simulink model "model_2023"  (R2023a)
settings: Solver=VariableStepAuto  StartTime=0.0  StopTime=100  RelTol=1e-3
settings Model: Creator=ian20030201  LastModifiedBy=ian20030201

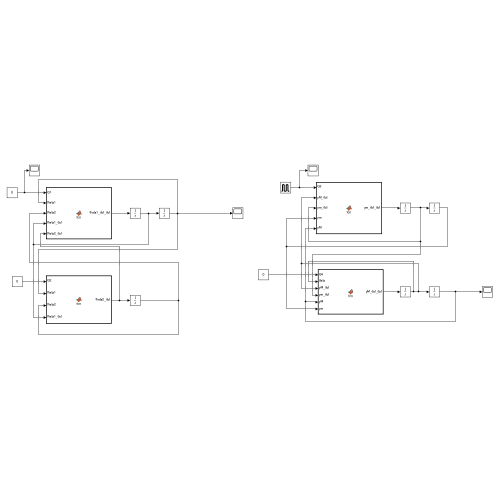
[thumbnail: Simulink's stored preview of the top-level diagram]
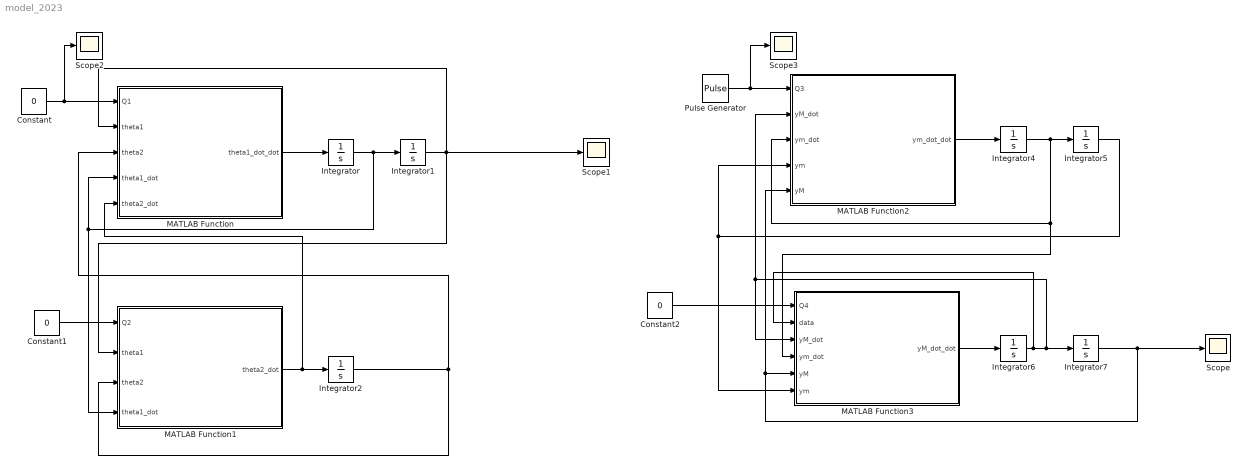
== system model_2023 ==
  Constant : Constant  Value=0
  Constant1 : Constant  Value=0
  Constant2 : Constant  Value=0
  Integrator{,1..2,4..7} (7 alike) : Integrator
  MATLAB Function : MATLAB Function  TreatAsAtomicUnit=on
  MATLAB Function1 : MATLAB Function  TreatAsAtomicUnit=on
  MATLAB Function2 : MATLAB Function  TreatAsAtomicUnit=on
  MATLAB Function3 : MATLAB Function  TreatAsAtomicUnit=on
  Pulse Generator : DiscretePulseGenerator  PulseType=Time based  Amplitude=20000  Period=100  PulseWidth=5  PhaseDelay=10
  Scope{,1..3} (4 alike) : Scope
  wires:
  MATLAB Function/1(theta1_dot_dot) -> Integrator/1
  Integrator/1 -> MATLAB Function1/4(theta1_dot), MATLAB Function/4(theta1_dot), Integrator1/1
  MATLAB Function1/1(theta2_dot) -> MATLAB Function/5(theta2_dot), Integrator2/1
  MATLAB Function2/1(ym_dot_dot) -> Integrator4/1
  Integrator4/1 -> MATLAB Function3/4(ym_dot), MATLAB Function2/3(ym_dot), Integrator5/1
  MATLAB Function3/1(yM_dot_dot) -> Integrator6/1
  Integrator6/1 -> MATLAB Function3/2(data), MATLAB Function3/3(yM_dot), MATLAB Function2/2(yM_dot), Integrator7/1
  Integrator2/1 -> MATLAB Function1/3(theta2), MATLAB Function/3(theta2)
  Integrator1/1 -> Scope1/1, MATLAB Function1/2(theta1), MATLAB Function/2(theta1)
  Integrator5/1 -> MATLAB Function3/6(ym), MATLAB Function2/4(ym)
  Integrator7/1 -> Scope/1, MATLAB Function2/5(yM), MATLAB Function3/5(yM)
  Constant/1 -> Scope2/1, MATLAB Function/1(Q1)
  Constant1/1 -> MATLAB Function1/1(Q2)
  Pulse Generator/1 -> Scope3/1, MATLAB Function2/1(Q3)
  Constant2/1 -> MATLAB Function3/1(Q4)

== matlab function model_2023/MATLAB Function1 ==
  data: Q2 input; theta2_dot output; theta1 input; theta2 input; theta1_dot input
function theta2_dot = fcn(Q2, theta1, theta2, theta1_dot)
c4 = 0.1;
l = 5;
k4 = 1000;
top = Q2 + c4 * l^2 * (cos(theta2) - cos(theta1 + theta2)) * cos(theta1 + theta2) * theta1_dot + k4 * l^2 * (sin(theta1 + 2*theta2) - 0.5 * sin(2*theta1 + 2*theta2) - 0.5 * sin(2*theta2));
bottom = c4 * l^2 * (cos(theta1 + theta2) - cos(theta2))^2;
bottom = 1;
theta2_dot = top / bottom;

== matlab function model_2023/MATLAB Function ==
  data: Q1 input; theta1_dot_dot output; theta1 input; theta2 input; theta1_dot input; theta2_dot input
function theta1_dot_dot = fcn(Q1, theta1, theta2, theta1_dot, theta2_dot)
c4 = 0.1;
l = 5;
m1 = 1000; m3 = 1000;
k1 = 1000; k3 = 1000; k4 = 1000;
g = 9.81;
top = Q1 - c4 * l^2 * (cos(theta1 + theta2))^2 * theta1_dot - c4 * l^2 * (cos(theta1 + theta2))^2 * theta2_dot + c4 * l^2 * (cos(theta1 + theta2)) * cos(theta2) * theta2_dot;
top = top - g * l * m1 * cos(theta1) + g * l * m3 * cos(theta1) - 0.5 * k1 * l^2 * sin(2*theta1) - 0.5 * k3 * l^2 * sin(2*theta1) - 0.5 * k4 * l^2 * sin(2*theta1) + 2 * theta2 + k4 * l^2 * sin(theta2) * cos(theta1 + theta2);
bottom = l^2 * (m1 + m3);

theta1_dot_dot = top / bottom;

== matlab function model_2023/MATLAB Function2 ==
  data: Q3 input; ym_dot_dot output; yM_dot input; ym_dot input; ym input; yM input
function ym_dot_dot = fcn(Q3, yM_dot, ym_dot, ym, yM)
theta_M = deg2rad(60);
M = 50; m2 = 10; m1 = 10; m3 = 10;
c5 = 100;
k2 = 500; k5 = 2000;
g = 9.81;
top = -M * g * (cos(theta_M))^2 - M * g + Q3 + c5 * (cos(theta_M))^2 * yM_dot - c5 * (cos(theta_M))^2 * ym_dot - g * m1 - g * m2 - g * m3 - k2 * ym + k5 * yM * (cos(theta_M))^2 - k5 * ym * (cos(theta_M))^2;
bottom = m2;

ym_dot_dot = top / bottom;

== matlab function model_2023/MATLAB Function3 ==
  data: Q4 input; data input; yM_dot_dot output; yM_dot input; ym_dot input; yM input; ym input
function yM_dot_dot = fcn(Q4, data, yM_dot, ym_dot, yM, ym)
theta_M = deg2rad(20);
M = 50;
c5 = 100;
k5 = 2000;
g = 9.81;
top = M * g * (cos(theta_M))^2 + Q4 - c5 * (cos(theta_M))^2 * yM_dot + c5 * (cos(theta_M))^2 * ym_dot - k5 * yM * (cos(theta_M))^2 + k5 * ym * (cos(theta_M))^2;
bottom = M;

yM_dot_dot = top / bottom;
